simulink model "Electric_Auto_simulink"  (R2024b)
settings: Solver=VariableStepAuto  StartTime=0.0  StopTime=100  RelTol=1e-3
values from neighbouring files (symbols this model uses):
  A_aero = 2.72    [Param_electric_auto.m]
  aw_acc = 1/Tau_acc    (= 0.993048659384)    [Param_electric_auto.m]
  beta1 = 0*pi/180    (= 0)    [Param_electric_auto.m]
  cR = 0.23    [Param_electric_auto.m]
  cW = 0.311    [Param_electric_auto.m]
  D = 0.8    [Param_electric_auto.m]
  deltaX_ref = VA_ref/2    (= 50)    [Param_electric_auto.m]
  F_B = 0    [Param_electric_auto.m]
  g = 9.81    [Param_electric_auto.m]
  i_g = 100    [Param_electric_auto.m]
  K_I = a_F*a_w/b_F    (= 0.0230278222222)    [Param_electric_auto.m]
  K_I_d = a_w_d*L_d    (= 0.136)    [Param_electric_auto.m]
  K_I_q = a_w_q*L_q    (= 0.136)    [Param_electric_auto.m]
  K_P = a_w/b_F    (= 4.76)    [Param_electric_auto.m]
  K_P_d = R_s*a_w_d    (= 2.88)    [Param_electric_auto.m]
  K_P_q = R_s*a_w_q    (= 2.88)    [Param_electric_auto.m]
  L_d = 0.0085    [Param_electric_auto.m]
  L_q = L_d    (= 0.0085)    [Param_electric_auto.m]
  m = m0 + delta_m    (= 2975)    [Param_electric_auto.m]
  Psi_PM = 0.0715    [Param_electric_auto.m]
  R_s = 0.18    [Param_electric_auto.m]
  Reff = 0.4    [Param_electric_auto.m]
  rho_air = 1.225    [Param_electric_auto.m]
  T_W = 300    [Param_electric_auto.m]
  V_B = 60    [Param_electric_auto.m]
  w_0 = 2    [Param_electric_auto.m]
  w_S = 30    [Param_electric_auto.m]
  XB_0 = 500    [Param_electric_auto.m]
  Z_p = 4    [Param_electric_auto.m]
settings Model: Creator=gille  LastModifiedBy=gille
settings RTWCC: GPUComputeCapability=3.5

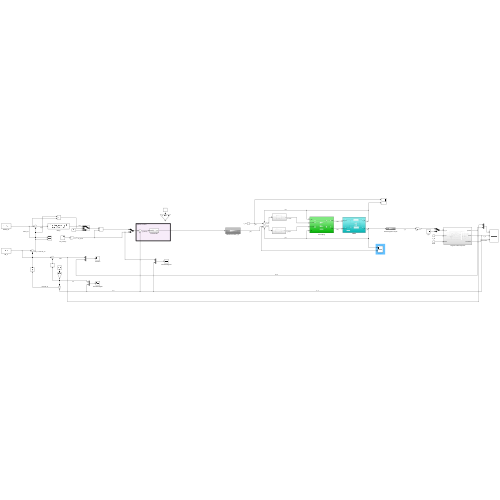
[thumbnail: Simulink's stored preview of the top-level diagram]
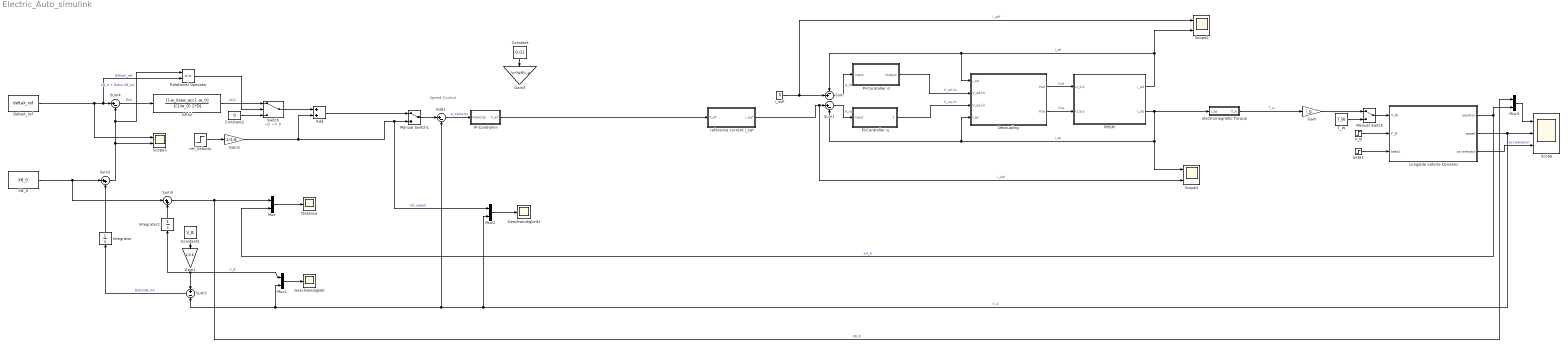
== system Electric_Auto_simulink ==
  note: Speed Control
  Add : Sum
  Add1 : Sum  Inputs=|+-
  Constant : Constant  Value=0.01
  Constant1 : Constant  Value=V_B
  Constant2 : Constant  Value=0
  Decoupling : Subsystem
  DeltaX_ref : Constant  Value=deltaX_ref
  Distance : Scope
  F_B : Step  After=F_B  SampleTime=0
  GR(s) : TransferFcn  Numerator=[(-w_0/aw_acc) -w_0]  Denominator=[(1/w_0) 2*D]
  Gain : Gain  Gain=i_g
  Gain1 : Gain  Gain=1/3.6
  Gain2 : Gain  Gain=1/3.6
  Gain3 : Gain  Gain=(m*Reff)/i_g
  Geschwindigkeit : Scope
  Geschwindigkeit1 : Scope
  Integrator : Integrator
  Integrator1 : Integrator
  Longside vehicle Dynamic : Subsystem
  Manual Switch : ManualSwitch
  Manual Switch1 : ManualSwitch
  Mux{,1..3} (4 alike) : Mux  Inputs=2
  PI-Controller : Subsystem
  PI-Controller d : Subsystem
  PI-Controller q : Subsystem
  PMSM : Subsystem
  Relational Operator : RelationalOperator  Operator=<=  OutDataTypeStr=boolean  RndMeth=Simplest  InputSameDT=off
  Scope : Scope  NumInputPorts=3
  Scope1 : Scope  NumInputPorts=2
  Scope2 : Scope  NumInputPorts=2
  Scope3 : Scope  NumInputPorts=2
  Sum : Sum  Inputs=-+|
  Sum1 : Sum  Inputs=|+-
  Sum2 : Sum  Inputs=|++
  Sum3 : Sum  Inputs=+-
  Sum4 : Sum  Inputs=|+-
  Sum5 : Sum  Inputs=|++
  Switch : Switch  Criteria=u2 ~= 0  SaturateOnIntegerOverflow=off  InputSameDT=off
  T_W : Constant  Value=T_W
  XB_0 : Constant  Value=XB_0
  beta1 : Step  After=beta1  SampleTime=0
  electromagnetic Torque : Subsystem
  i_sd* : Constant  Value=0
  ref_Velocity : Step  After=100  SampleTime=0
  reference current i_sq* : Subsystem
  wires:
  Longside vehicle Dynamic/2(speed) -> Scope/2, Mux2/2, Add1/2, Mux1/2, Sum3/2  "V_A"
  Longside vehicle Dynamic/3(accelerator) -> Scope/3  "acceleration"
  F_B/1 -> Longside vehicle Dynamic/2(F_B)
  beta1/1 -> Longside vehicle Dynamic/3(beta1)
  T_W/1 -> Manual Switch/2
  Manual Switch/1 -> Longside vehicle Dynamic/1(T_W)
  ref_Velocity/1 -> Gain2/1
  Sum1/1 -> PI-Controller q/1(Input)  "e_iq"
  i_sd*/1 -> Sum/2, Scope2/1  "i_sd*"
  reference current i_sq*/1(i_sq*) -> Scope1/2, Sum1/1  "i_sq*"
  Sum/1 -> PI-Controller d/1(Input)  "e_id"
  Manual Switch1/1 -> Add1/1
  Gain2/1 -> Add/2, Manual Switch1/2, Mux2/1  "ref_speed"
  PMSM/1(i_sd) -> Sum/1, Decoupling/1(i_sd), Scope2/2  "i_sd"
  PMSM/2(i_sq) -> Scope1/1, Sum1/2, Decoupling/4(i_qs), electromagnetic Torque/1(i_qs)  "i_sq"
  PI-Controller d/1(Output) -> Decoupling/2(V_sd,lin)  "V_sd,lin"
  PI-Controller q/1(1) -> Decoupling/3(V_sq,lin)  "V_sq,lin"
  Decoupling/1(Vsd) -> PMSM/1(U_S,d)  "Vsd"
  Decoupling/2(Vsq) -> PMSM/2(U_S,q)  "Vsq"
  PI-Controller/1(T_e*) -> reference current i_sq*/1(T_e*)
  Constant/1 -> Gain3/1
  Add1/1 -> PI-Controller/1(Velocity)  "e_Velocity"
  GR(s)/1 -> Switch/1  "U(s)"
  Sum4/1 -> GR(s)/1  "E(s)"
  Add/1 -> Manual Switch1/1
  Constant1/1 -> Gain1/1
  Gain1/1 -> Sum3/1, Mux1/1, Integrator1/1  "V_B"
  Sum3/1 -> Integrator/1  "DeltaVB_VA"
  Gain/1 -> Manual Switch/1
  electromagnetic Torque/1(T_e) -> Gain/1  "T_e"
  Integrator/1 -> Sum2/2
  Sum2/1 -> Scope3/2, Relational Operator/1, Sum4/2  "XB_0 + Delta VB_VA"
  DeltaX_ref/1 -> Scope3/1, Relational Operator/2, Sum4/1  "DeltaX_ref"
  Switch/1 -> Add/1
  Constant2/1 -> Switch/3
  Relational Operator/1 -> Switch/2
  Integrator1/1 -> Sum5/2
  XB_0/1 -> Sum2/1, Sum5/1
  Sum5/1 -> Mux/1, Mux3/1  "XB_0"
  Longside vehicle Dynamic/1(position) -> Mux3/2, Mux/2  "XA_0"
  Mux/1 -> Distance/1
  Mux1/1 -> Geschwindigkeit/1
  Mux2/1 -> Geschwindigkeit1/1
  Mux3/1 -> Scope/1

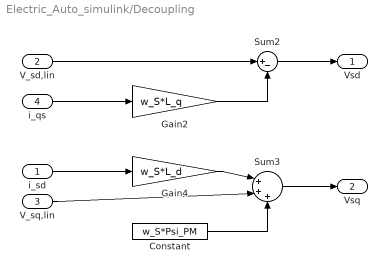
== system Electric_Auto_simulink/Decoupling ==
  i_sd : Inport
  V_sd,lin : Inport  Port=2
  V_sq,lin : Inport  Port=3
  i_qs : Inport  Port=4
  Constant : Constant  Value=w_S*Psi_PM
  Gain2 : Gain  Gain=w_S*L_q
  Gain4 : Gain  Gain=w_S*L_d
  Sum2 : Sum  Inputs=|+-
  Sum3 : Sum  Inputs=|+++
  Vsd : Outport
  Vsq : Outport  Port=2
  wires:
  Sum3/1 -> Vsq/1
  Gain2/1 -> Sum2/2
  V_sd,lin/1 -> Sum2/1
  i_sd/1 -> Gain4/1
  Gain4/1 -> Sum3/1
  i_qs/1 -> Gain2/1
  Constant/1 -> Sum3/3
  V_sq,lin/1 -> Sum3/2
  Sum2/1 -> Vsd/1

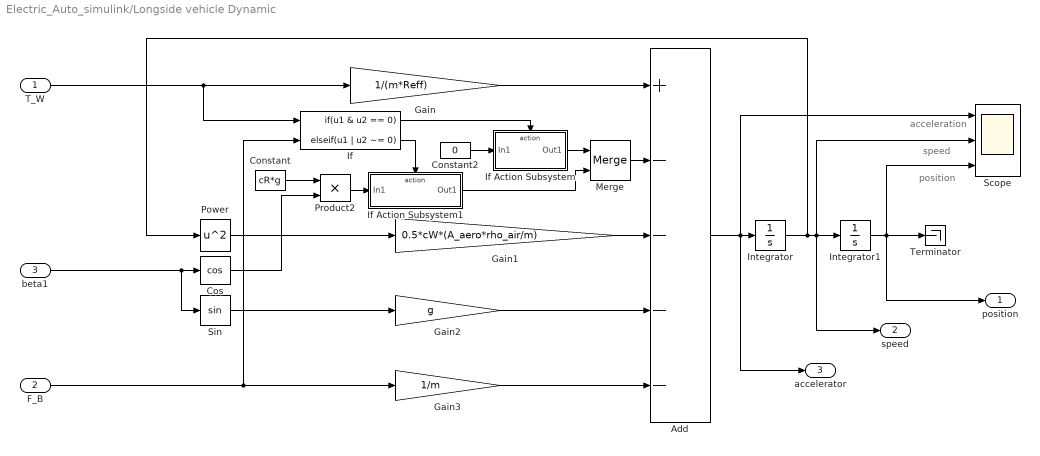
== system Electric_Auto_simulink/Longside vehicle Dynamic ==
  note: position
  note: speed
  note: acceleration
  T_W : Inport
  F_B : Inport  Port=2
  beta1 : Inport  Port=3
  Add : Sum  Inputs=+----
  Constant : Constant  Value=cR*g
  Constant2 : Constant  Value=0
  Cos : Trigonometry  Operator=cos
  Gain : Gain  Gain=1/(m*Reff)
  Gain1 : Gain  Gain=0.5*cW*(A_aero*rho_air/m)
  Gain2 : Gain  Gain=g
  Gain3 : Gain  Gain=1/m
  If : If  NumInputs=2  IfExpression=u1 & u2 == 0  ElseIfExpressions=u1 | u2 ~= 0  ShowElse=off
  If Action Subsystem : Subsystem  TreatAsAtomicUnit=on
  If Action Subsystem1 : Subsystem  TreatAsAtomicUnit=on
  Integrator : Integrator
  Integrator1 : Integrator
  Merge : Merge
  Power : Math  Operator=square
  Product2 : Product
  Scope : Scope  NumInputPorts=3
  Sin : Trigonometry
  Terminator : Terminator
  position : Outport
  speed : Outport  Port=2
  accelerator : Outport  Port=3
  wires:
  Add/1 -> Scope/1, Integrator/1, accelerator/1
  Constant/1 -> Product2/1
  Power/1 -> Gain1/1
  beta1/1 -> Sin/1, Cos/1
  Gain2/1 -> Add/4
  F_B/1 -> If/2, Gain3/1
  If/2 -> If Action Subsystem1/Action
  T_W/1 -> Gain/1, If/1
  Product2/1 -> If Action Subsystem1/1(In1)
  Sin/1 -> Gain2/1
  Integrator/1 -> Power/1, Integrator1/1, speed/1, Scope/2
  Gain/1 -> Add/1
  Integrator1/1 -> Terminator/1, position/1, Scope/3
  If Action Subsystem/1(Out1) -> Merge/1
  If/1 -> If Action Subsystem/Action
  Constant2/1 -> If Action Subsystem/1(In1)
  Gain3/1 -> Add/5
  Cos/1 -> Product2/2
  If Action Subsystem1/1(Out1) -> Merge/2
  Merge/1 -> Add/2
  Gain1/1 -> Add/3

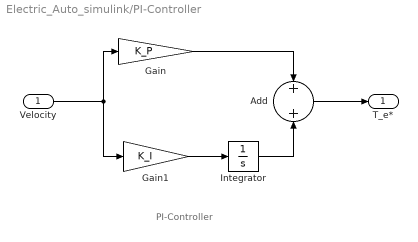
== system Electric_Auto_simulink/PI-Controller ==
  note: PI-Controller
  Velocity : Inport
  Add : Sum
  Gain : Gain  Gain=K_P
  Gain1 : Gain  Gain=K_I
  Integrator : Integrator
  T_e* : Outport
  wires:
  Gain/1 -> Add/1
  Gain1/1 -> Integrator/1
  Integrator/1 -> Add/2
  Add/1 -> T_e*/1
  Velocity/1 -> Gain1/1, Gain/1

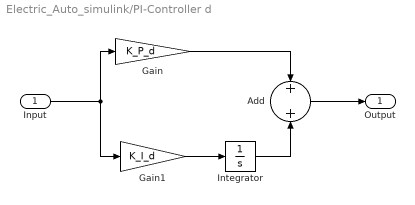
== system Electric_Auto_simulink/PI-Controller d ==
  Input : Inport
  Add : Sum
  Gain : Gain  Gain=K_P_d
  Gain1 : Gain  Gain=K_I_d
  Integrator : Integrator
  Output : Outport
  wires:
  Gain/1 -> Add/1
  Gain1/1 -> Integrator/1
  Integrator/1 -> Add/2
  Add/1 -> Output/1
  Input/1 -> Gain1/1, Gain/1

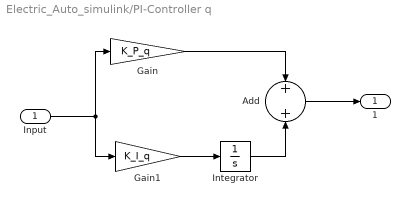
== system Electric_Auto_simulink/PI-Controller q ==
  Input : Inport
  Add : Sum
  Gain : Gain  Gain=K_P_q
  Gain1 : Gain  Gain=K_I_q
  Integrator : Integrator
  1 : Outport
  wires:
  Gain/1 -> Add/1
  Gain1/1 -> Integrator/1
  Integrator/1 -> Add/2
  Add/1 -> 1/1
  Input/1 -> Gain1/1, Gain/1

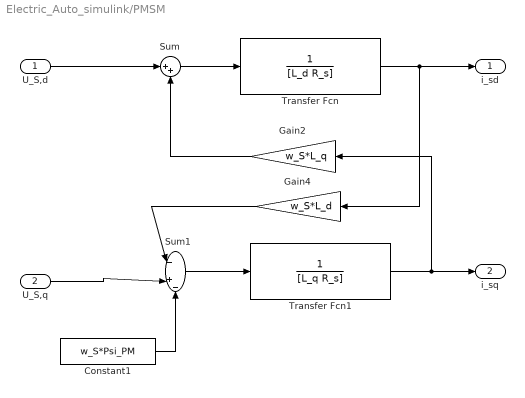
== system Electric_Auto_simulink/PMSM ==
  U_S,d : Inport
  U_S,q : Inport  Port=2
  Constant1 : Constant  Value=w_S*Psi_PM
  Gain2 : Gain  Gain=w_S*L_q
  Gain4 : Gain  Gain=w_S*L_d
  Sum : Sum  Inputs=|++
  Sum1 : Sum  Inputs=|-+-
  Transfer Fcn : TransferFcn  Denominator=[L_d R_s]
  Transfer Fcn1 : TransferFcn  Denominator=[L_q R_s]
  i_sd : Outport
  i_sq : Outport  Port=2
  wires:
  U_S,d/1 -> Sum/1
  Sum/1 -> Transfer Fcn/1
  Gain2/1 -> Sum/2
  Transfer Fcn/1 -> Gain4/1, i_sd/1
  Constant1/1 -> Sum1/3
  U_S,q/1 -> Sum1/2
  Gain4/1 -> Sum1/1
  Sum1/1 -> Transfer Fcn1/1
  Transfer Fcn1/1 -> Gain2/1, i_sq/1

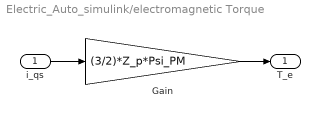
== system Electric_Auto_simulink/electromagnetic Torque ==
  i_qs : Inport
  Gain : Gain  Gain=(3/2)*Z_p*Psi_PM
  T_e : Outport
  wires:
  Gain/1 -> T_e/1
  i_qs/1 -> Gain/1

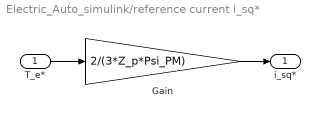
== system Electric_Auto_simulink/reference current i_sq* ==
  T_e* : Inport
  Gain : Gain  Gain=2/(3*Z_p*Psi_PM)
  i_sq* : Outport
  wires:
  Gain/1 -> i_sq*/1
  T_e*/1 -> Gain/1

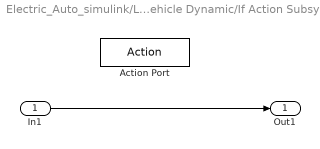
== system Electric_Auto_simulink/Longside vehicle Dynamic/If Action Subsystem ==
  In1 : Inport
  Action Port : ActionPort  ActionPortLabel=if(u1 & u2 == 0)
  Out1 : Outport
  wires:
  In1/1 -> Out1/1

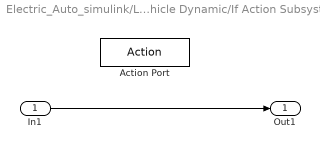
== system Electric_Auto_simulink/Longside vehicle Dynamic/If Action Subsystem1 ==
  In1 : Inport
  Action Port : ActionPort  ActionPortLabel=elseif(u1 | u2 ~= 0)
  Out1 : Outport
  wires:
  In1/1 -> Out1/1
